simulink model "RefModel_complementary"  (R2020a)
settings: Solver=ode1  StartTime=0.0  StopTime=10.0  FixedStep=Ts_Navi.Ts_Base  RelTol=1e-3
libraries: aerolibgravity2 x1
settings Model: Creator=computer  LastModifiedBy=computer

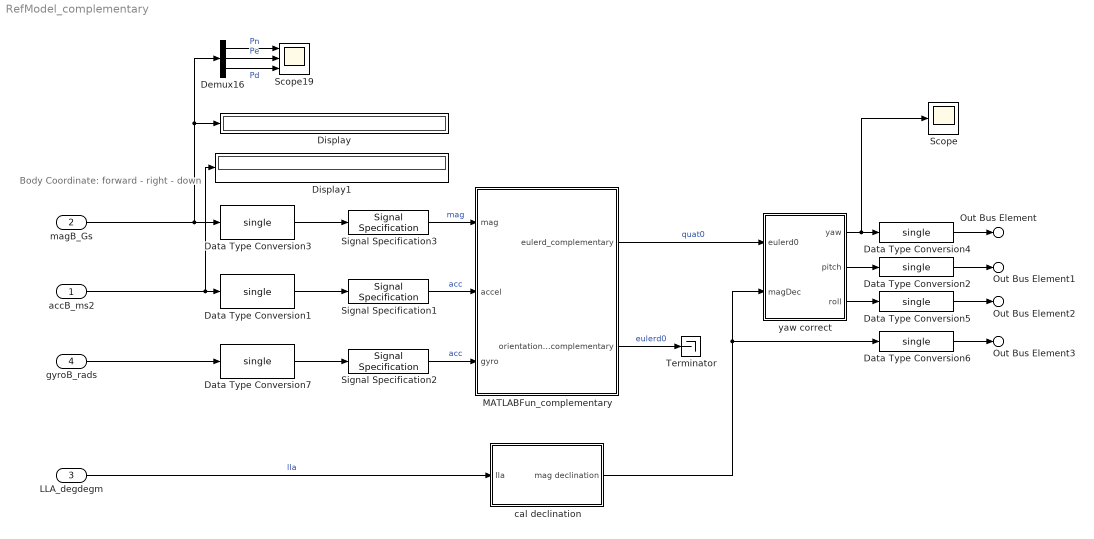
== system RefModel_complementary ==
  note: Body Coordinate: forward - right - down
  accB_ms2 : Inport  PortDimensions=[1,3]
  magB_Gs : Inport  Port=2  PortDimensions=[1,3]
  LLA_degdegm : Inport  Port=3  PortDimensions=[1,3]
  gyroB_rads : Inport  Port=4  PortDimensions=[1,3]
  Data Type Conversion{1..7} (7 alike) : DataTypeConversion  OutDataTypeStr=single
  Demux16 : Demux  Outputs=3
  Display : Display
  Display1 : Display
  MATLABFun_complementary : MATLAB Function  TreatAsAtomicUnit=on
  Scope : Scope
  Scope19 : Scope  NumInputPorts=3
  Signal Specification1 : SignalSpecification  Dimensions=[1,3]
  Signal Specification2 : SignalSpecification  Dimensions=[1,3]
  Signal Specification3 : SignalSpecification  Dimensions=[1,3]
  Terminator : Terminator
  cal declination : Subsystem
  yaw correct : Subsystem
  Out Bus Element : Outport  PortName=complementary_out  Element=compass_yawd
  Out Bus Element1 : Outport  PortName=complementary_out  Element=compass_pitchd
  Out Bus Element2 : Outport  PortName=complementary_out  Element=compass_rolld
  Out Bus Element3 : Outport  PortName=complementary_out  Element=compass_magDeclinationd
  wires:
  Data Type Conversion2/1 -> Out Bus Element1/1
  Data Type Conversion3/1 -> Signal Specification3/1
  Demux16/1 -> Scope19/1  "Pn"
  Data Type Conversion6/1 -> Out Bus Element3/1
  Signal Specification3/1 -> MATLABFun_complementary/1(mag)  "mag"
  yaw correct/2(pitch) -> Data Type Conversion2/1
  Demux16/2 -> Scope19/2  "Pe"
  Data Type Conversion5/1 -> Out Bus Element2/1
  Signal Specification1/1 -> MATLABFun_complementary/2(accel)  "acc"
  cal declination/1(mag declination) -> Data Type Conversion6/1, yaw correct/2(magDec)
  yaw correct/1(yaw) -> Scope/1, Data Type Conversion4/1
  yaw correct/3(roll) -> Data Type Conversion5/1
  Data Type Conversion4/1 -> Out Bus Element/1
  LLA_degdegm/1 -> cal declination/1(lla)  "lla"
  Data Type Conversion1/1 -> Signal Specification1/1
  accB_ms2/1 -> Display1/1, Data Type Conversion1/1
  magB_Gs/1 -> Demux16/1, Display/1, Data Type Conversion3/1
  Demux16/3 -> Scope19/3  "Pd"
  Data Type Conversion7/1 -> Signal Specification2/1
  gyroB_rads/1 -> Data Type Conversion7/1
  Signal Specification2/1 -> MATLABFun_complementary/3(gyro)  "acc"
  MATLABFun_complementary/1(eulerd_complementary) -> yaw correct/1(eulerd0)  "quat0"
  MATLABFun_complementary/2(orientation_complementary) -> Terminator/1  "eulerd0"

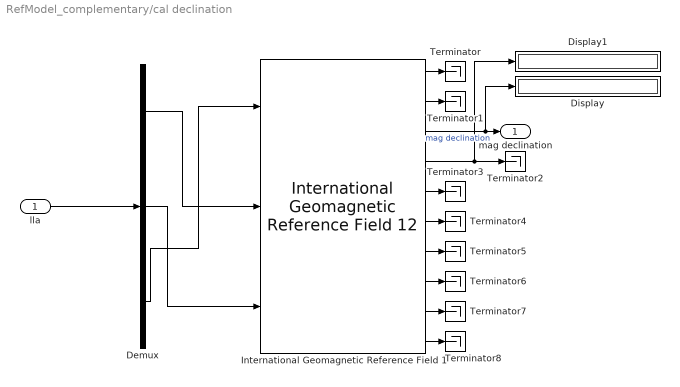
== system RefModel_complementary/cal declination ==
  lla : Inport
  Demux : Demux  Outputs=3
  Display : Display
  Display1 : Display
  International Geomagnetic Reference Field 1 : aerolibgravity2/International Geomagnetic Reference Field 12  units=Metric (MKS)  time_in=off  month=January  day=1  year=2020  action=None  sv_out=on
      settings: SourceProductBaseCode=AE
  Terminator{,1..8} (9 alike) : Terminator
  mag declination : Outport
  wires:
  Demux/3 -> International Geomagnetic Reference Field 1/1
  Demux/1 -> International Geomagnetic Reference Field 1/2
  International Geomagnetic Reference Field 1/9 -> Terminator7/1
  International Geomagnetic Reference Field 1/10 -> Terminator8/1
  International Geomagnetic Reference Field 1/4 -> Display1/1, Terminator2/1
  International Geomagnetic Reference Field 1/1 -> Terminator/1
  Demux/2 -> International Geomagnetic Reference Field 1/3
  International Geomagnetic Reference Field 1/2 -> Terminator1/1
  International Geomagnetic Reference Field 1/3 -> Display/1, mag declination/1  "mag declination"
  International Geomagnetic Reference Field 1/5 -> Terminator3/1
  International Geomagnetic Reference Field 1/6 -> Terminator4/1
  International Geomagnetic Reference Field 1/8 -> Terminator6/1
  International Geomagnetic Reference Field 1/7 -> Terminator5/1
  lla/1 -> Demux/1

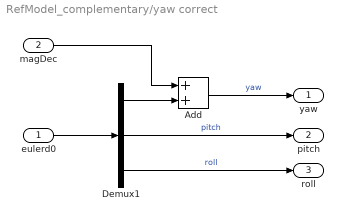
== system RefModel_complementary/yaw correct ==
  eulerd0 : Inport
  magDec : Inport  Port=2
  Add : Sum
  Demux1 : Demux  Outputs=3
  yaw : Outport
  pitch : Outport  Port=2
  roll : Outport  Port=3
  wires:
  magDec/1 -> Add/1
  eulerd0/1 -> Demux1/1
  Demux1/2 -> pitch/1  "pitch"
  Demux1/3 -> roll/1  "roll"
  Demux1/1 -> Add/2
  Add/1 -> yaw/1  "yaw"

== matlab function RefModel_complementary/MATLABFun_complementary ==
  data: eulerd_complementary output; mag input; accel input; orientation_complementary output; gyro input
function [eulerd_complementary,orientation_complementary] = complementary(mag,accel, gyro)
persistent filter_complementary orientation_complementary0
if isempty(filter_complementary)
    % Complementary
    filter_complementary = complementaryFilter;
    filter_complementary.SampleRate = 1000/12;
    orientation_complementary0 = [1,0,0,0];
end
%% Complementary
if ~all(accel==0)
    orientation_complementary = compact(filter_complementary(double(accel),double(gyro),double(mag)));
else
    orientation_complementary = orientation_complementary0;
end
eulerd_complementary = double(eulerd(orientation_complementary));
orientation_complementary0 = orientation_complementary;
end


function eout = eulerd(quat)
% rotate 'ZYX'
qa = quat(1);
qb = quat(2);
qc = quat(3);
qd = quat(4);
the1 = single(1);
the2 = single(2);

tmp = qb.*qd.*the2 - qa.*qc.*the2;
if tmp > the1
    tmp = the1;
elseif tmp < -the1
    tmp = -the1;
end
% tmp(tmp > the1) = the1;
% tmp(tmp < -the1) = -the1;
b = -asin(tmp);
a = atan2((qa.*qd.*the2 + qb.*qc.*the2),(qa.^2.*the2 - the1 + qb.^2.*the2));
c = atan2((qa.*qb.*the2 + qc.*qd.*the2),(qa.^2.*the2 - the1 + qd.^2.*the2));
eout = [a b c]*180/pi;
end

%
% function [eulerd0,quat0] = compass(i,accel,mag,imuUpdateFs,magUpdateFs)
%     fs = imuUpdateFs;
%     quat0 = zeros(1,4);
%     eulerd0 = zeros(1,3);
%     if rem(i,fs/magUpdateFs) == 0 && i ~= 1
%         quat0 = compact(ecompass(accel,mag));
%         eulerd0 = eulerd(quat0);
%     end
% end
